simulink model "Controller_Designation_Simul_PD"  (R2025a)
settings: Solver=ode4  StartTime=Tstart  StopTime=Tend  FixedStep=Tsim  RelTol=1e-3
values from neighbouring files (symbols this model uses):
  Gm_den = [1 31.1403]    [Controller_Designation_Design.m]    (also in Controller_Designation_Pole_Placement.m; Controller_Designation_Simulation.m = [1 1/tau_m])
  Gm_num = [10.88]    [Controller_Designation_Design.m]    (also in Controller_Designation_Pole_Placement.m; Controller_Designation_Simulation.m = [Km/tau_m])
  Kd = (tau_m * 2 * wn * zeta - 1) / (Km * Kg)    [Controller_Designation_Design.m]    (also in Controller_Designation_Pole_Placement.m; Controller_Designation_Simulation.m = 0.00117352840074)
  Kg = 1/0.00067    (= 1492.53731343)    [Controller_Designation_Design.m]    (also in Controller_Designation_Pole_Placement.m; Controller_Designation_Simulation.m)
  Kp = (wn^2 * tau_m) / (Km * Kg)    [Controller_Designation_Design.m]    (also in Controller_Designation_Pole_Placement.m; Controller_Designation_Simulation.m = 0.0776073069853)
  Ts = 0.005    [Controller_Designation_Simulation.m]
  Tsim = 0.001    [Controller_Designation_Simulation.m]
settings Model: Creator=Ryuminseo  LastModifiedBy=Ryuminseo

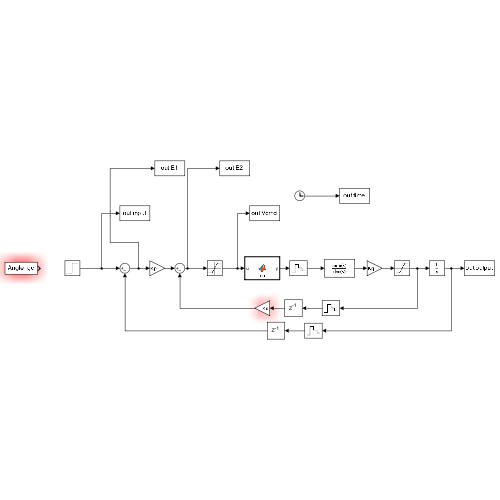
[thumbnail: Simulink's stored preview of the top-level diagram]
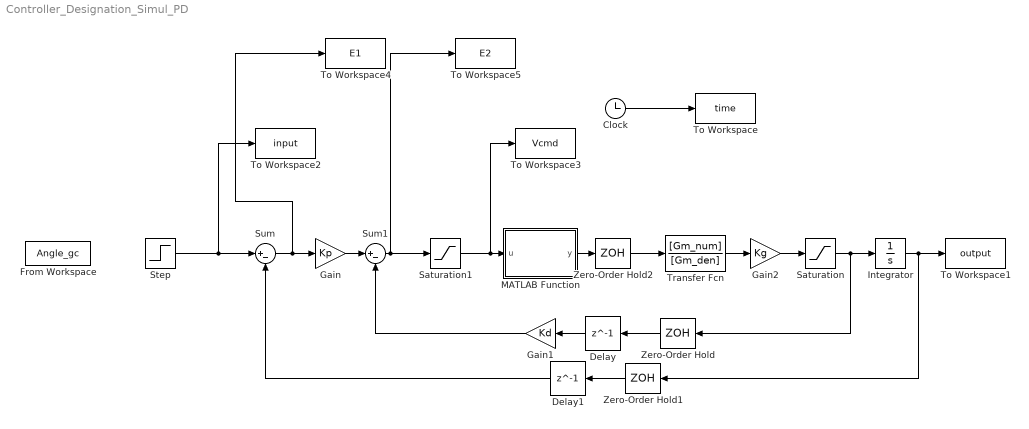
== system Controller_Designation_Simul_PD ==
  Clock : Clock
  Delay : Delay  DelayLength=1  InitialCondition=0  SampleTime=Ts
  Delay1 : Delay  DelayLength=1  InitialCondition=0  SampleTime=Ts
  From Workspace : FromWorkspace  VariableName=Angle_gc
  Gain : Gain  Gain=Kp
  Gain1 : Gain  Gain=Kd
  Gain2 : Gain  Gain=Kg
  Integrator : Integrator
  MATLAB Function : MATLAB Function  TreatAsAtomicUnit=on
  Saturation : Saturate  UpperLimit=1200  LowerLimit=-1200
  Saturation1 : Saturate  UpperLimit=2.5  LowerLimit=-2.5
  Step : Step  Time=0  After=20  SampleTime=Ts
  Sum : Sum  Inputs=|+-
  Sum1 : Sum  Inputs=|+-
  To Workspace : ToWorkspace  VariableName=time  SampleTime=-1
  To Workspace1 : ToWorkspace  VariableName=output  SampleTime=Tsim
  To Workspace2 : ToWorkspace  VariableName=input  SampleTime=Tsim
  To Workspace3 : ToWorkspace  VariableName=Vcmd  SampleTime=Tsim
  To Workspace4 : ToWorkspace  VariableName=E1  SampleTime=Tsim
  To Workspace5 : ToWorkspace  VariableName=E2  SampleTime=Tsim
  Transfer Fcn : TransferFcn  Numerator=[Gm_num]  Denominator=[Gm_den]
  Zero-Order Hold : ZeroOrderHold  SampleTime=Ts
  Zero-Order Hold1 : ZeroOrderHold  SampleTime=Ts
  Zero-Order Hold2 : ZeroOrderHold  SampleTime=Ts
  wires:
  Transfer Fcn/1 -> Gain2/1
  Clock/1 -> To Workspace/1
  Sum/1 -> To Workspace4/1, Gain/1
  Integrator/1 -> To Workspace1/1, Zero-Order Hold1/1
  Delay1/1 -> Sum/2
  Delay/1 -> Gain1/1
  Gain2/1 -> Saturation/1
  Saturation/1 -> Zero-Order Hold/1, Integrator/1
  Zero-Order Hold/1 -> Delay/1
  Zero-Order Hold1/1 -> Delay1/1
  Zero-Order Hold2/1 -> Transfer Fcn/1
  Gain/1 -> Sum1/1
  Sum1/1 -> Saturation1/1, To Workspace5/1
  MATLAB Function/1(y) -> Zero-Order Hold2/1
  Saturation1/1 -> To Workspace3/1, MATLAB Function/1(u)
  Step/1 -> To Workspace2/1, Sum/1
  Gain1/1 -> Sum1/2

== matlab function Controller_Designation_Simul_PD/MATLAB Function ==
  data: u input; y output
function y = fcn(u)

    if u >= -0.1 && u <= 0.1
        y = 0;
        
    else
        y = u;
    end
end
